simulink library "Simscape_Bit_Multiplexers_Lib"  (R2023a)
settings: Solver=ode45  StartTime=0.0  StopTime=10.0  RelTol=1e-3  EnableMultiTasking=on
libraries: Simscape_Gates_Lib x11
settings Model: Creator=uzivatel  LastModifiedBy=Jozko Mrkvicka
settings SolverCC: AlgebraicLoopSolver=TrustRegion
settings DataIOCC: LimitDataPoints=on  SaveFormat=Array  ReturnWorkspaceOutputs=off
settings OptimizationCC: LifeSpan=inf
settings DebuggingCC: UnderspecifiedInitializationDetection=Classic  MergeDetectMultiDrivingBlocksExec=none  SolverPrmCheckMsg=warning  UnconnectedInputMsg=warning  UnconnectedOutputMsg=warning  UnconnectedLineMsg=warning  StateNameClashWarn=warning  SFUnexpectedBacktrackingDiag=warning  SFNoUnconditionalDefaultTransitionDiag=warning  ArithmeticOperatorsInVariantConditions=warning
settings HardwareCC: ProdBitPerPointer=32  ProdBitPerSizeT=32  ProdBitPerPtrDiffT=32  ProdLargestAtomicFloat=None  ProdIntDivRoundTo=Undefined  ProdEndianess=Unspecified  ProdWordSize=32  ProdHWDeviceType=32-bit Generic
settings ModelReferenceCC: EnableRefExpFcnMdlSchedulingChecks=on  PropagateSignalLabelsOutOfModel=off
settings SFSimCC: SimUseLocalCustomCode=off  CustomCodeUndefinedFunction=UseInterfaceOnly
settings RTWCC: RTWUseLocalCustomCode=off
settings CodeAppCC: StateflowObjectComments=on
settings GRTTargetCC: TargetLangStandard=C89/C90 (ANSI)
settings ConfigComp: CovMetricSettings=dw  CovSaveCumulativeToWorkspaceVar=on  CovSaveSingleToWorkspaceVar=on  CovExternalEMLEnable=off

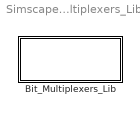
== system Simscape_Bit_Multiplexers_Lib ==
  Bit_Multiplexers_Lib : Subsystem

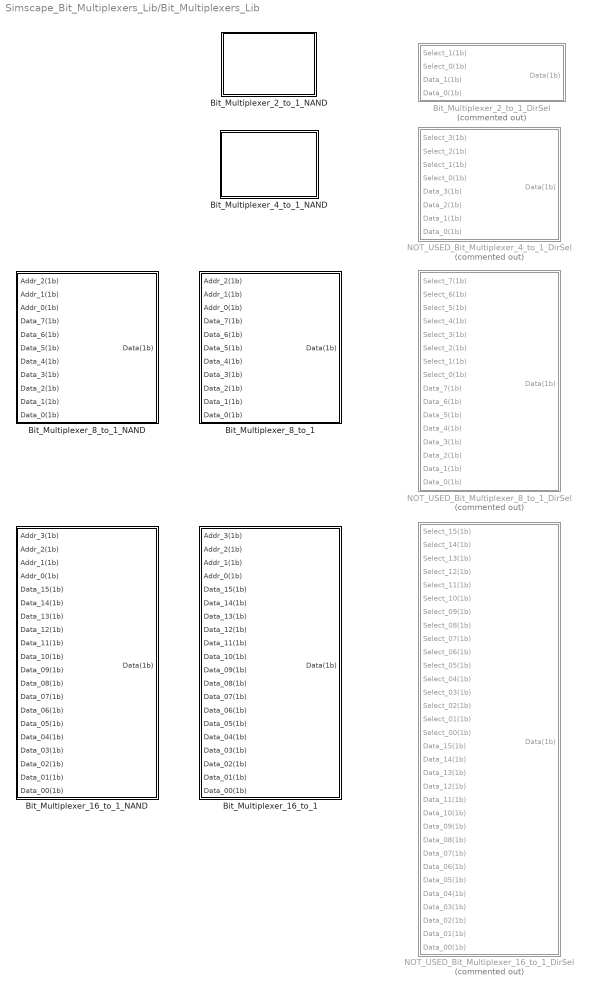
== system Simscape_Bit_Multiplexers_Lib/Bit_Multiplexers_Lib ==
  Bit_Multiplexer_16_to_1 : Subsystem
  Bit_Multiplexer_16_to_1_NAND : Subsystem
  Bit_Multiplexer_2_to_1_DirSel : Subsystem  Commented=on
  Bit_Multiplexer_2_to_1_NAND : Subsystem
      settings: PortSchema="{\"entries\":[{\"content\":{\"sides\":[{\"content\":{\"connectorIds\":[\"LConn1\",\"LConn2\",\"LConn3\"]},\"type\":\"ConnectorPlacement.EquallySpacedRectSide\",\"uuid\":\"05aa9ed7-c40b-4846-b9c5-a59fe7474fe7\"},{\"content\":{\"connectorIds\":[\"RConn1\"],\"side\":\"RIGHT\"},\"type\":\"ConnectorPlacement.EquallySpacedRectSide\",\"uuid\":\"f4c26865-c23f-4e2d-9b22-f32510006689\"},{\"content\":{\"connectorIds\":[\"LConn4\"],\"side\":\"TOP\"},\"type\":\"ConnectorPlacement.EquallySpacedRectSide\",\"uuid\":\"5ca9bb1e-e0f6-480e-8c02-f26cf148a313\"},{\"content\":{\"connectorIds\":[\"RConn2\"],\"side\":\"BOTTOM\"},\"type\":\"ConnectorPlacement.EquallySpacedRectSide\",\"uuid\":\"bd4becbe-1bbd-422f-b22f-c30d52f9b7b5\"}]},\"type\":\"ConnectorPlacement.EquallySpacedConnector\",\"uuid\":\"13373c58-d26b-438c-b680-b1e730634329\"}],\"packageUris\":[\"http://schema.mathworks.com/mf0/Connector/R2020b\"],\"version\":\"1.0\"}"
  Bit_Multiplexer_4_to_1_NAND : Subsystem
      settings: PortSchema="{\"entries\":[{\"content\":{\"sides\":[{\"content\":{\"connectorIds\":[\"LConn1\",\"LConn2\",\"LConn3\",\"LConn4\",\"LConn5\",\"LConn6\"]},\"type\":\"ConnectorPlacement.EquallySpacedRectSide\",\"uuid\":\"05aa9ed7-c40b-4846-b9c5-a59fe7474fe7\"},{\"content\":{\"connectorIds\":[\"RConn1\"],\"side\":\"RIGHT\"},\"type\":\"ConnectorPlacement.EquallySpacedRectSide\",\"uuid\":\"f4c26865-c23f-4e2d-9b22-f32510006689\"},{\"content\":{\"connectorIds\":[\"LConn7\"],\"side\":\"TOP\"},\"type\":\"ConnectorPlacement.EquallySpacedRectSide\",\"uuid\":\"5ca9bb1e-e0f6-480e-8c02-f26cf148a313\"},{\"content\":{\"connectorIds\":[\"RConn2\"],\"side\":\"BOTTOM\"},\"type\":\"ConnectorPlacement.EquallySpacedRectSide\",\"uuid\":\"bd4becbe-1bbd-422f-b22f-c30d52f9b7b5\"}]},\"type\":\"ConnectorPlacement.EquallySpacedConnector\",\"uuid\":\"13373c58-d26b-438c-b680-b1e730634329\"}],\"packageUris\":[\"http://schema.mathworks.com/mf0/Connector/R2020b\"],\"version\":\"1.0\"}"
  Bit_Multiplexer_8_to_1 : Subsystem
  Bit_Multiplexer_8_to_1_NAND : Subsystem
  NOT_USED_Bit_Multiplexer_16_to_1_DirSel : Subsystem  Commented=on
  NOT_USED_Bit_Multiplexer_4_to_1_DirSel : Subsystem  Commented=on
  NOT_USED_Bit_Multiplexer_8_to_1_DirSel : Subsystem  Commented=on

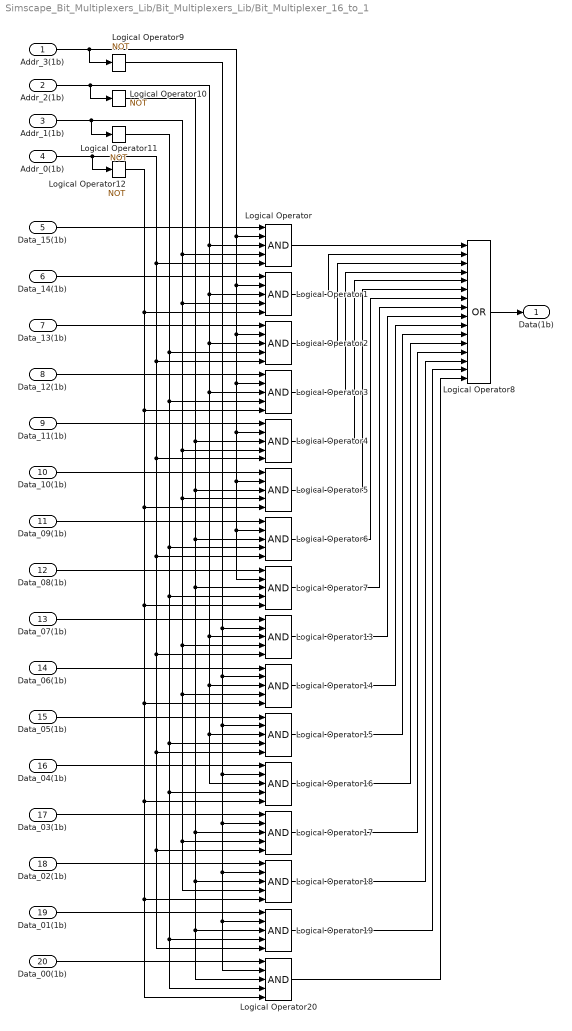
== system Simscape_Bit_Multiplexers_Lib/Bit_Multiplexers_Lib/Bit_Multiplexer_16_to_1 ==
  Addr_3(1b) : Inport
  Addr_2(1b) : Inport  Port=2
  Addr_1(1b) : Inport  Port=3
  Addr_0(1b) : Inport  Port=4
  Data_15(1b) : Inport  Port=5
  Data_14(1b) : Inport  Port=6
  Data_13(1b) : Inport  Port=7
  Data_12(1b) : Inport  Port=8
  Data_11(1b) : Inport  Port=9
  Data_10(1b) : Inport  Port=10
  Data_09(1b) : Inport  Port=11
  Data_08(1b) : Inport  Port=12
  Data_07(1b) : Inport  Port=13
  Data_06(1b) : Inport  Port=14
  Data_05(1b) : Inport  Port=15
  Data_04(1b) : Inport  Port=16
  Data_03(1b) : Inport  Port=17
  Data_02(1b) : Inport  Port=18
  Data_01(1b) : Inport  Port=19
  Data_00(1b) : Inport  Port=20
  Logical Operator{,1..7,13..20} (16 alike) : Logic  Inputs=5  IconShape=distinctive  AllPortsSameDT=off  OutDataTypeStr=boolean
  Logical Operator{9..12} (4 alike) : Logic  Operator=NOT  Inputs=4  IconShape=distinctive  AllPortsSameDT=off  OutDataTypeStr=boolean
  Logical Operator8 : Logic  Operator=OR  Inputs=16  IconShape=distinctive  OutDataTypeStr=boolean
  Data(1b) : Outport
  wires:
  Logical Operator12/1 -> Logical Operator20/5, Logical Operator18/5, Logical Operator16/5, Logical Operator14/5, Logical Operator7/5, Logical Operator5/5, Logical Operator3/5, Logical Operator1/5
  Addr_0(1b)/1 -> Logical Operator15/5, Logical Operator17/5, Logical Operator19/5, Logical Operator13/5, Logical Operator6/5, Logical Operator4/5, Logical Operator2/5, Logical Operator/5, Logical Operator12/1
  Logical Operator11/1 -> Logical Operator20/4, Logical Operator19/4, Logical Operator16/4, Logical Operator15/4, Logical Operator7/4, Logical Operator6/4, Logical Operator3/4, Logical Operator2/4
  Addr_1(1b)/1 -> Logical Operator18/4, Logical Operator17/4, Logical Operator14/4, Logical Operator13/4, Logical Operator5/4, Logical Operator4/4, Logical Operator1/4, Logical Operator/4, Logical Operator11/1
  Logical Operator10/1 -> Logical Operator20/3, Logical Operator19/3, Logical Operator18/3, Logical Operator17/3, Logical Operator7/3, Logical Operator6/3, Logical Operator5/3, Logical Operator4/3
  Addr_2(1b)/1 -> Logical Operator16/3, Logical Operator15/3, Logical Operator14/3, Logical Operator13/3, Logical Operator3/3, Logical Operator2/3, Logical Operator1/3, Logical Operator/3, Logical Operator10/1
  Logical Operator9/1 -> Logical Operator20/2, Logical Operator19/2, Logical Operator18/2, Logical Operator17/2, Logical Operator16/2, Logical Operator15/2, Logical Operator14/2, Logical Operator13/2
  Addr_3(1b)/1 -> Logical Operator3/2, Logical Operator4/2, Logical Operator7/2, Logical Operator6/2, Logical Operator5/2, Logical Operator2/2, Logical Operator1/2, Logical Operator/2, Logical Operator9/1
  Data_00(1b)/1 -> Logical Operator20/1
  Data_01(1b)/1 -> Logical Operator19/1
  Data_02(1b)/1 -> Logical Operator18/1
  Data_03(1b)/1 -> Logical Operator17/1
  Data_04(1b)/1 -> Logical Operator16/1
  Data_05(1b)/1 -> Logical Operator15/1
  Data_06(1b)/1 -> Logical Operator14/1
  Data_07(1b)/1 -> Logical Operator13/1
  Logical Operator20/1 -> Logical Operator8/16
  Logical Operator19/1 -> Logical Operator8/15
  Logical Operator18/1 -> Logical Operator8/14
  Logical Operator17/1 -> Logical Operator8/13
  Logical Operator16/1 -> Logical Operator8/12
  Logical Operator15/1 -> Logical Operator8/11
  Logical Operator14/1 -> Logical Operator8/10
  Logical Operator13/1 -> Logical Operator8/9
  Logical Operator8/1 -> Data(1b)/1
  Data_15(1b)/1 -> Logical Operator/1
  Data_14(1b)/1 -> Logical Operator1/1
  Data_13(1b)/1 -> Logical Operator2/1
  Data_12(1b)/1 -> Logical Operator3/1
  Data_11(1b)/1 -> Logical Operator4/1
  Data_10(1b)/1 -> Logical Operator5/1
  Data_09(1b)/1 -> Logical Operator6/1
  Data_08(1b)/1 -> Logical Operator7/1
  Logical Operator7/1 -> Logical Operator8/8
  Logical Operator6/1 -> Logical Operator8/7
  Logical Operator5/1 -> Logical Operator8/6
  Logical Operator4/1 -> Logical Operator8/5
  Logical Operator3/1 -> Logical Operator8/4
  Logical Operator2/1 -> Logical Operator8/3
  Logical Operator1/1 -> Logical Operator8/2
  Logical Operator/1 -> Logical Operator8/1

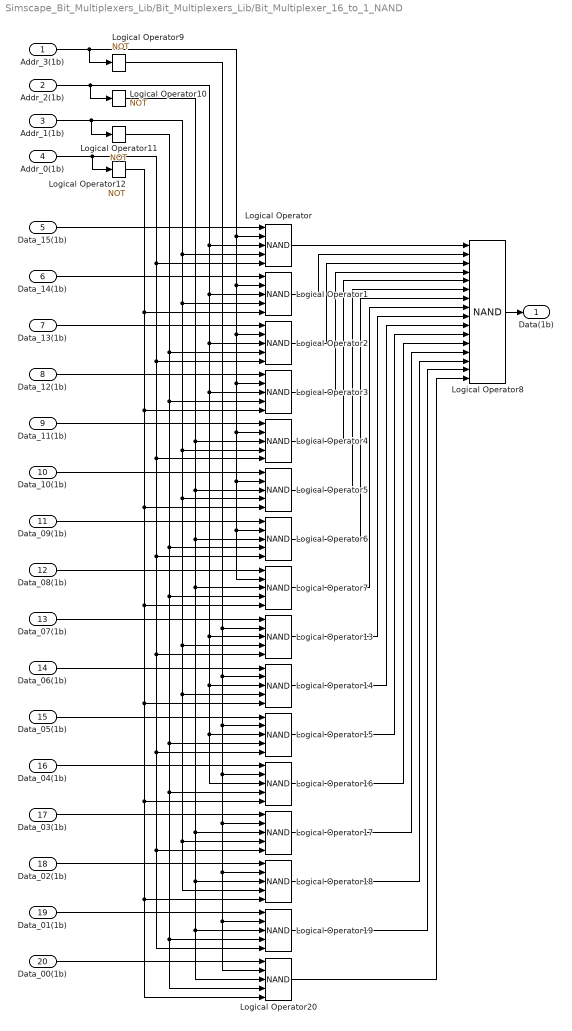
== system Simscape_Bit_Multiplexers_Lib/Bit_Multiplexers_Lib/Bit_Multiplexer_16_to_1_NAND ==
  Addr_3(1b) : Inport
  Addr_2(1b) : Inport  Port=2
  Addr_1(1b) : Inport  Port=3
  Addr_0(1b) : Inport  Port=4
  Data_15(1b) : Inport  Port=5
  Data_14(1b) : Inport  Port=6
  Data_13(1b) : Inport  Port=7
  Data_12(1b) : Inport  Port=8
  Data_11(1b) : Inport  Port=9
  Data_10(1b) : Inport  Port=10
  Data_09(1b) : Inport  Port=11
  Data_08(1b) : Inport  Port=12
  Data_07(1b) : Inport  Port=13
  Data_06(1b) : Inport  Port=14
  Data_05(1b) : Inport  Port=15
  Data_04(1b) : Inport  Port=16
  Data_03(1b) : Inport  Port=17
  Data_02(1b) : Inport  Port=18
  Data_01(1b) : Inport  Port=19
  Data_00(1b) : Inport  Port=20
  Logical Operator{,1..7,13..20} (16 alike) : Logic  Operator=NAND  Inputs=5  IconShape=distinctive  AllPortsSameDT=off  OutDataTypeStr=boolean
  Logical Operator{9..12} (4 alike) : Logic  Operator=NOT  Inputs=4  IconShape=distinctive  AllPortsSameDT=off  OutDataTypeStr=boolean
  Logical Operator8 : Logic  Operator=NAND  Inputs=16  IconShape=distinctive  OutDataTypeStr=boolean
  Data(1b) : Outport
  wires:
  Logical Operator12/1 -> Logical Operator20/5, Logical Operator18/5, Logical Operator16/5, Logical Operator14/5, Logical Operator7/5, Logical Operator5/5, Logical Operator3/5, Logical Operator1/5
  Addr_0(1b)/1 -> Logical Operator15/5, Logical Operator17/5, Logical Operator19/5, Logical Operator13/5, Logical Operator6/5, Logical Operator4/5, Logical Operator2/5, Logical Operator/5, Logical Operator12/1
  Logical Operator11/1 -> Logical Operator20/4, Logical Operator19/4, Logical Operator16/4, Logical Operator15/4, Logical Operator7/4, Logical Operator6/4, Logical Operator3/4, Logical Operator2/4
  Addr_1(1b)/1 -> Logical Operator18/4, Logical Operator17/4, Logical Operator14/4, Logical Operator13/4, Logical Operator5/4, Logical Operator4/4, Logical Operator1/4, Logical Operator/4, Logical Operator11/1
  Logical Operator10/1 -> Logical Operator20/3, Logical Operator19/3, Logical Operator18/3, Logical Operator17/3, Logical Operator7/3, Logical Operator6/3, Logical Operator5/3, Logical Operator4/3
  Addr_2(1b)/1 -> Logical Operator16/3, Logical Operator15/3, Logical Operator14/3, Logical Operator13/3, Logical Operator3/3, Logical Operator2/3, Logical Operator1/3, Logical Operator/3, Logical Operator10/1
  Logical Operator9/1 -> Logical Operator20/2, Logical Operator19/2, Logical Operator18/2, Logical Operator17/2, Logical Operator16/2, Logical Operator15/2, Logical Operator14/2, Logical Operator13/2
  Addr_3(1b)/1 -> Logical Operator3/2, Logical Operator4/2, Logical Operator7/2, Logical Operator6/2, Logical Operator5/2, Logical Operator2/2, Logical Operator1/2, Logical Operator/2, Logical Operator9/1
  Data_00(1b)/1 -> Logical Operator20/1
  Data_01(1b)/1 -> Logical Operator19/1
  Data_02(1b)/1 -> Logical Operator18/1
  Data_03(1b)/1 -> Logical Operator17/1
  Data_04(1b)/1 -> Logical Operator16/1
  Data_05(1b)/1 -> Logical Operator15/1
  Data_06(1b)/1 -> Logical Operator14/1
  Data_07(1b)/1 -> Logical Operator13/1
  Logical Operator20/1 -> Logical Operator8/16
  Logical Operator19/1 -> Logical Operator8/15
  Logical Operator18/1 -> Logical Operator8/14
  Logical Operator17/1 -> Logical Operator8/13
  Logical Operator16/1 -> Logical Operator8/12
  Logical Operator15/1 -> Logical Operator8/11
  Logical Operator14/1 -> Logical Operator8/10
  Logical Operator13/1 -> Logical Operator8/9
  Logical Operator8/1 -> Data(1b)/1
  Data_15(1b)/1 -> Logical Operator/1
  Data_14(1b)/1 -> Logical Operator1/1
  Data_13(1b)/1 -> Logical Operator2/1
  Data_12(1b)/1 -> Logical Operator3/1
  Data_11(1b)/1 -> Logical Operator4/1
  Data_10(1b)/1 -> Logical Operator5/1
  Data_09(1b)/1 -> Logical Operator6/1
  Data_08(1b)/1 -> Logical Operator7/1
  Logical Operator7/1 -> Logical Operator8/8
  Logical Operator6/1 -> Logical Operator8/7
  Logical Operator5/1 -> Logical Operator8/6
  Logical Operator4/1 -> Logical Operator8/5
  Logical Operator3/1 -> Logical Operator8/4
  Logical Operator2/1 -> Logical Operator8/3
  Logical Operator1/1 -> Logical Operator8/2
  Logical Operator/1 -> Logical Operator8/1

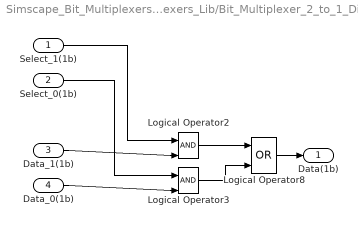
== system Simscape_Bit_Multiplexers_Lib/Bit_Multiplexers_Lib/Bit_Multiplexer_2_to_1_DirSel ==
  Select_1(1b) : Inport
  Select_0(1b) : Inport  Port=2
  Data_1(1b) : Inport  Port=3
  Data_0(1b) : Inport  Port=4
  Logical Operator2 : Logic  IconShape=distinctive  AllPortsSameDT=off  OutDataTypeStr=boolean
  Logical Operator3 : Logic  IconShape=distinctive  AllPortsSameDT=off  OutDataTypeStr=boolean
  Logical Operator8 : Logic  Operator=OR  IconShape=distinctive  OutDataTypeStr=boolean
  Data(1b) : Outport
  wires:
  Logical Operator8/1 -> Data(1b)/1
  Logical Operator3/1 -> Logical Operator8/2
  Logical Operator2/1 -> Logical Operator8/1
  Data_1(1b)/1 -> Logical Operator2/2
  Data_0(1b)/1 -> Logical Operator3/2
  Select_1(1b)/1 -> Logical Operator2/1
  Select_0(1b)/1 -> Logical Operator3/1

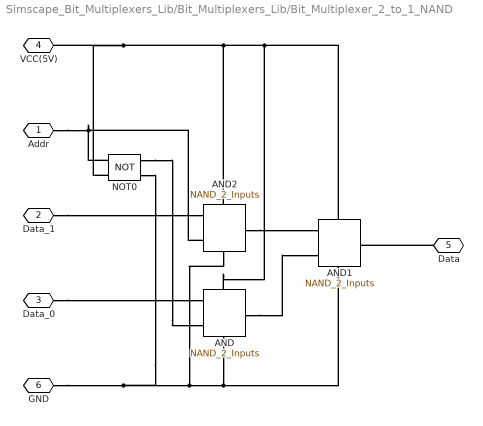
== system Simscape_Bit_Multiplexers_Lib/Bit_Multiplexers_Lib/Bit_Multiplexer_2_to_1_NAND ==
  AND : Simscape_Gates_Lib/NAND_2_Inputs  SystemSampleTime=-1  VariantActivationTime=update diagram  Latency=0  AutoFrameSizeCalculation=off
      settings: LibrarySourceBlock=pokus_lib/AND  PortSchema="{\"entries\":[{\"content\":{\"sides\":[{\"content\":{\"connectorIds\":[\"LConn1\",\"LConn2\"]},\"type\":\"ConnectorPlacement.EquallySpacedRectSide\",\"uuid\":\"1f677ca5-ee16-40a0-87d2-2e95da8c7721\"},{\"content\":{\"connectorIds\":[\"RConn1\"],\"side\":\"RIGHT\"},\"type\":\"ConnectorPlacement.EquallySpacedRectSide\",\"uuid\":\"f9e7d437-b89a-4416-b804-8f11fd927687\"},{\"content\":{\"connectorIds\":[\"LConn3\"],\"side\":\"TOP\"},\"type\":\"ConnectorPlacement.EquallySpacedRectSide\",\"uuid\":\"bd4824ff-3399-4fe5-aaaa-59980d9198b6\"},{\"content\":{\"connectorIds\":[\"RConn2\"],\"side\":\"BOTTOM\"},\"type\":\"ConnectorPlacement.EquallySpacedRectSide\",\"uuid\":\"eafb0998-9a7e-4634-b7fa-91494491415c\"}]},\"type\":\"ConnectorPlacement.EquallySpacedConnector\",\"uuid\":\"9f76a3c8-f141-459c-8f30-1ffa838c3ea4\"}],\"packageUris\":[\"http://schema.mathworks.com/mf0/Connector/R2020b\"],\"version\":\"1.0\"}"
  AND1 : Simscape_Gates_Lib/NAND_2_Inputs  SystemSampleTime=-1  VariantActivationTime=update diagram  Latency=0  AutoFrameSizeCalculation=off
      settings: LibrarySourceBlock=pokus_lib/AND  PortSchema="{\"entries\":[{\"content\":{\"sides\":[{\"content\":{\"connectorIds\":[\"LConn1\",\"LConn2\"]},\"type\":\"ConnectorPlacement.EquallySpacedRectSide\",\"uuid\":\"1f677ca5-ee16-40a0-87d2-2e95da8c7721\"},{\"content\":{\"connectorIds\":[\"RConn1\"],\"side\":\"RIGHT\"},\"type\":\"ConnectorPlacement.EquallySpacedRectSide\",\"uuid\":\"f9e7d437-b89a-4416-b804-8f11fd927687\"},{\"content\":{\"connectorIds\":[\"LConn3\"],\"side\":\"TOP\"},\"type\":\"ConnectorPlacement.EquallySpacedRectSide\",\"uuid\":\"bd4824ff-3399-4fe5-aaaa-59980d9198b6\"},{\"content\":{\"connectorIds\":[\"RConn2\"],\"side\":\"BOTTOM\"},\"type\":\"ConnectorPlacement.EquallySpacedRectSide\",\"uuid\":\"eafb0998-9a7e-4634-b7fa-91494491415c\"}]},\"type\":\"ConnectorPlacement.EquallySpacedConnector\",\"uuid\":\"9f76a3c8-f141-459c-8f30-1ffa838c3ea4\"}],\"packageUris\":[\"http://schema.mathworks.com/mf0/Connector/R2020b\"],\"version\":\"1.0\"}"
  AND2 : Simscape_Gates_Lib/NAND_2_Inputs  SystemSampleTime=-1  VariantActivationTime=update diagram  Latency=0  AutoFrameSizeCalculation=off
      settings: LibrarySourceBlock=pokus_lib/AND  PortSchema="{\"entries\":[{\"content\":{\"sides\":[{\"content\":{\"connectorIds\":[\"LConn1\",\"LConn2\"]},\"type\":\"ConnectorPlacement.EquallySpacedRectSide\",\"uuid\":\"1f677ca5-ee16-40a0-87d2-2e95da8c7721\"},{\"content\":{\"connectorIds\":[\"RConn1\"],\"side\":\"RIGHT\"},\"type\":\"ConnectorPlacement.EquallySpacedRectSide\",\"uuid\":\"f9e7d437-b89a-4416-b804-8f11fd927687\"},{\"content\":{\"connectorIds\":[\"LConn3\"],\"side\":\"TOP\"},\"type\":\"ConnectorPlacement.EquallySpacedRectSide\",\"uuid\":\"bd4824ff-3399-4fe5-aaaa-59980d9198b6\"},{\"content\":{\"connectorIds\":[\"RConn2\"],\"side\":\"BOTTOM\"},\"type\":\"ConnectorPlacement.EquallySpacedRectSide\",\"uuid\":\"eafb0998-9a7e-4634-b7fa-91494491415c\"}]},\"type\":\"ConnectorPlacement.EquallySpacedConnector\",\"uuid\":\"9f76a3c8-f141-459c-8f30-1ffa838c3ea4\"}],\"packageUris\":[\"http://schema.mathworks.com/mf0/Connector/R2020b\"],\"version\":\"1.0\"}"
  NOT0 : Simscape_Gates_Lib/NOT
  Addr : PMIOPort  Side=Left
  Data_1 : PMIOPort  Port=2  Side=Left
  Data_0 : PMIOPort  Port=3  Side=Left
  VCC(5V) : PMIOPort  Port=4  Side=Left
  Data : PMIOPort  Port=5  Side=Right
  GND : PMIOPort  Port=6  Side=Right
  connections:
  VCC(5V)/RConn1 -- AND2/LConn3 -- AND1/LConn3 -- AND/LConn3 -- NOT0/LConn2
  Data_0/RConn1 -- AND/LConn1
  Data_1/RConn1 -- AND2/LConn1
  NOT0/RConn1 -- AND/LConn2
  AND2/RConn1 -- AND1/LConn1
  AND/RConn1 -- AND1/LConn2
  Data/RConn1 -- AND1/RConn1
  AND2/LConn2 -- Addr/RConn1 -- NOT0/LConn1
  AND/RConn2 -- AND1/RConn2 -- AND2/RConn2 -- GND/RConn1 -- NOT0/RConn2

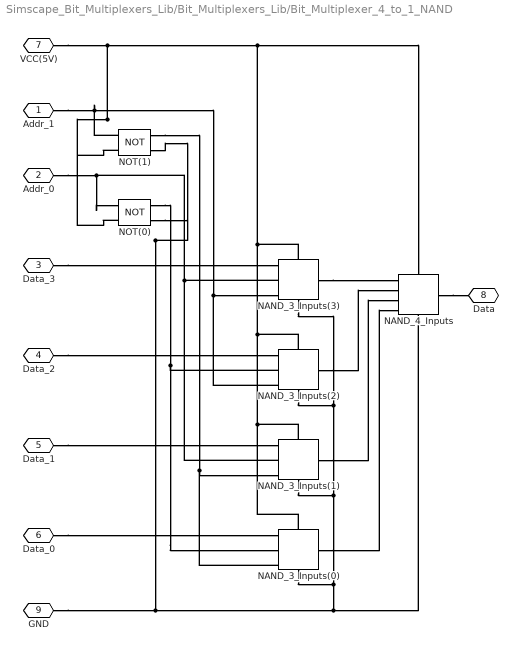
== system Simscape_Bit_Multiplexers_Lib/Bit_Multiplexers_Lib/Bit_Multiplexer_4_to_1_NAND ==
  NAND_3_Inputs(0) : Simscape_Gates_Lib/NAND_3_Inputs  SystemSampleTime=-1  VariantActivationTime=update diagram  Latency=0  AutoFrameSizeCalculation=off
      settings: PortSchema="{\"entries\":[{\"content\":{\"sides\":[{\"content\":{\"connectorIds\":[\"LConn1\",\"LConn2\",\"LConn3\"]},\"type\":\"ConnectorPlacement.EquallySpacedRectSide\",\"uuid\":\"3ad033e8-f540-4908-b767-0851e4a6512c\"},{\"content\":{\"connectorIds\":[\"RConn1\"],\"side\":\"RIGHT\"},\"type\":\"ConnectorPlacement.EquallySpacedRectSide\",\"uuid\":\"66ead7bd-a472-46db-941e-d4ec7399d328\"},{\"content\":{\"connectorIds\":[\"LConn4\"],\"side\":\"TOP\"},\"type\":\"ConnectorPlacement.EquallySpacedRectSide\",\"uuid\":\"cb3c8fc5-feff-4b6f-b91b-692680a0eeb1\"},{\"content\":{\"connectorIds\":[\"RConn2\"],\"side\":\"BOTTOM\"},\"type\":\"ConnectorPlacement.EquallySpacedRectSide\",\"uuid\":\"f8b8aaf7-b6fc-45dd-a5cf-24360dfeaf9c\"}]},\"type\":\"ConnectorPlacement.EquallySpacedConnector\",\"uuid\":\"2d561a3f-f784-4d92-a395-6823d790bdb8\"}],\"packageUris\":[\"http://schema.mathworks.com/mf0/Connector/R2020b\"],\"version\":\"1.0\"}"
  NAND_3_Inputs(1) : Simscape_Gates_Lib/NAND_3_Inputs  SystemSampleTime=-1  VariantActivationTime=update diagram  Latency=0  AutoFrameSizeCalculation=off
      settings: PortSchema="{\"entries\":[{\"content\":{\"sides\":[{\"content\":{\"connectorIds\":[\"LConn1\",\"LConn2\",\"LConn3\"]},\"type\":\"ConnectorPlacement.EquallySpacedRectSide\",\"uuid\":\"3ad033e8-f540-4908-b767-0851e4a6512c\"},{\"content\":{\"connectorIds\":[\"RConn1\"],\"side\":\"RIGHT\"},\"type\":\"ConnectorPlacement.EquallySpacedRectSide\",\"uuid\":\"66ead7bd-a472-46db-941e-d4ec7399d328\"},{\"content\":{\"connectorIds\":[\"LConn4\"],\"side\":\"TOP\"},\"type\":\"ConnectorPlacement.EquallySpacedRectSide\",\"uuid\":\"cb3c8fc5-feff-4b6f-b91b-692680a0eeb1\"},{\"content\":{\"connectorIds\":[\"RConn2\"],\"side\":\"BOTTOM\"},\"type\":\"ConnectorPlacement.EquallySpacedRectSide\",\"uuid\":\"f8b8aaf7-b6fc-45dd-a5cf-24360dfeaf9c\"}]},\"type\":\"ConnectorPlacement.EquallySpacedConnector\",\"uuid\":\"2d561a3f-f784-4d92-a395-6823d790bdb8\"}],\"packageUris\":[\"http://schema.mathworks.com/mf0/Connector/R2020b\"],\"version\":\"1.0\"}"
  NAND_3_Inputs(2) : Simscape_Gates_Lib/NAND_3_Inputs  SystemSampleTime=-1  VariantActivationTime=update diagram  Latency=0  AutoFrameSizeCalculation=off
      settings: PortSchema="{\"entries\":[{\"content\":{\"sides\":[{\"content\":{\"connectorIds\":[\"LConn1\",\"LConn2\",\"LConn3\"]},\"type\":\"ConnectorPlacement.EquallySpacedRectSide\",\"uuid\":\"3ad033e8-f540-4908-b767-0851e4a6512c\"},{\"content\":{\"connectorIds\":[\"RConn1\"],\"side\":\"RIGHT\"},\"type\":\"ConnectorPlacement.EquallySpacedRectSide\",\"uuid\":\"66ead7bd-a472-46db-941e-d4ec7399d328\"},{\"content\":{\"connectorIds\":[\"LConn4\"],\"side\":\"TOP\"},\"type\":\"ConnectorPlacement.EquallySpacedRectSide\",\"uuid\":\"cb3c8fc5-feff-4b6f-b91b-692680a0eeb1\"},{\"content\":{\"connectorIds\":[\"RConn2\"],\"side\":\"BOTTOM\"},\"type\":\"ConnectorPlacement.EquallySpacedRectSide\",\"uuid\":\"f8b8aaf7-b6fc-45dd-a5cf-24360dfeaf9c\"}]},\"type\":\"ConnectorPlacement.EquallySpacedConnector\",\"uuid\":\"2d561a3f-f784-4d92-a395-6823d790bdb8\"}],\"packageUris\":[\"http://schema.mathworks.com/mf0/Connector/R2020b\"],\"version\":\"1.0\"}"
  NAND_3_Inputs(3) : Simscape_Gates_Lib/NAND_3_Inputs  SystemSampleTime=-1  VariantActivationTime=update diagram  Latency=0  AutoFrameSizeCalculation=off
      settings: PortSchema="{\"entries\":[{\"content\":{\"sides\":[{\"content\":{\"connectorIds\":[\"LConn1\",\"LConn2\",\"LConn3\"]},\"type\":\"ConnectorPlacement.EquallySpacedRectSide\",\"uuid\":\"3ad033e8-f540-4908-b767-0851e4a6512c\"},{\"content\":{\"connectorIds\":[\"RConn1\"],\"side\":\"RIGHT\"},\"type\":\"ConnectorPlacement.EquallySpacedRectSide\",\"uuid\":\"66ead7bd-a472-46db-941e-d4ec7399d328\"},{\"content\":{\"connectorIds\":[\"LConn4\"],\"side\":\"TOP\"},\"type\":\"ConnectorPlacement.EquallySpacedRectSide\",\"uuid\":\"cb3c8fc5-feff-4b6f-b91b-692680a0eeb1\"},{\"content\":{\"connectorIds\":[\"RConn2\"],\"side\":\"BOTTOM\"},\"type\":\"ConnectorPlacement.EquallySpacedRectSide\",\"uuid\":\"f8b8aaf7-b6fc-45dd-a5cf-24360dfeaf9c\"}]},\"type\":\"ConnectorPlacement.EquallySpacedConnector\",\"uuid\":\"2d561a3f-f784-4d92-a395-6823d790bdb8\"}],\"packageUris\":[\"http://schema.mathworks.com/mf0/Connector/R2020b\"],\"version\":\"1.0\"}"
  NAND_4_Inputs : Simscape_Gates_Lib/NAND_4_Inputs  SystemSampleTime=-1  VariantActivationTime=update diagram  Latency=0  AutoFrameSizeCalculation=off
      settings: PortSchema="{\"entries\":[{\"content\":{\"sides\":[{\"content\":{\"connectorIds\":[\"LConn1\",\"LConn2\",\"LConn3\",\"LConn4\"]},\"type\":\"ConnectorPlacement.EquallySpacedRectSide\",\"uuid\":\"4919ea86-d7f6-40d9-8c6d-90ddc4d67a92\"},{\"content\":{\"connectorIds\":[\"RConn1\"],\"side\":\"RIGHT\"},\"type\":\"ConnectorPlacement.EquallySpacedRectSide\",\"uuid\":\"1df2866f-d4b5-4a77-86de-714a74631175\"},{\"content\":{\"connectorIds\":[\"LConn5\"],\"side\":\"TOP\"},\"type\":\"ConnectorPlacement.EquallySpacedRectSide\",\"uuid\":\"d2ff5589-d2f7-4904-bc04-37eddab71799\"},{\"content\":{\"connectorIds\":[\"RConn2\"],\"side\":\"BOTTOM\"},\"type\":\"ConnectorPlacement.EquallySpacedRectSide\",\"uuid\":\"d97c62b3-511d-41ae-a18a-ca90ba3cee24\"}]},\"type\":\"ConnectorPlacement.EquallySpacedConnector\",\"uuid\":\"361286e1-4e89-40b7-926b-afe9d68e3bc9\"}],\"packageUris\":[\"http://schema.mathworks.com/mf0/Connector/R2020b\"],\"version\":\"1.0\"}"
  NOT(0) : Simscape_Gates_Lib/NOT
  NOT(1) : Simscape_Gates_Lib/NOT
  Addr_1 : PMIOPort  Side=Left
  Addr_0 : PMIOPort  Port=2  Side=Left
  Data_3 : PMIOPort  Port=3  Side=Left
  Data_2 : PMIOPort  Port=4  Side=Left
  Data_1 : PMIOPort  Port=5  Side=Left
  Data_0 : PMIOPort  Port=6  Side=Left
  VCC(5V) : PMIOPort  Port=7  Side=Left
  Data : PMIOPort  Port=8  Side=Right
  GND : PMIOPort  Port=9  Side=Right
  connections:
  NAND_4_Inputs/RConn1 -- Data/RConn1
  NAND_3_Inputs(3)/RConn1 -- NAND_4_Inputs/LConn1
  NAND_3_Inputs(2)/RConn1 -- NAND_4_Inputs/LConn2
  NAND_3_Inputs(1)/RConn1 -- NAND_4_Inputs/LConn3
  NAND_3_Inputs(0)/RConn1 -- NAND_4_Inputs/LConn4
  NOT(0)/RConn1 -- NAND_3_Inputs(2)/LConn2 -- NAND_3_Inputs(0)/LConn2
  NAND_3_Inputs(3)/LConn2 -- NAND_3_Inputs(1)/LConn2 -- NOT(0)/LConn1 -- Addr_0/RConn1
  Addr_1/RConn1 -- NOT(1)/LConn1 -- NAND_3_Inputs(3)/LConn3 -- NAND_3_Inputs(2)/LConn3
  NOT(1)/RConn1 -- NAND_3_Inputs(1)/LConn3 -- NAND_3_Inputs(0)/LConn3
  Data_3/RConn1 -- NAND_3_Inputs(3)/LConn1
  Data_2/RConn1 -- NAND_3_Inputs(2)/LConn1
  Data_1/RConn1 -- NAND_3_Inputs(1)/LConn1
  Data_0/RConn1 -- NAND_3_Inputs(0)/LConn1
  VCC(5V)/RConn1 -- NOT(0)/LConn2 -- NOT(1)/LConn2 -- NAND_3_Inputs(0)/LConn4 -- NAND_3_Inputs(1)/LConn4 -- NAND_3_Inputs(2)/LConn4 -- NAND_3_Inputs(3)/LConn4 -- NAND_4_Inputs/LConn5
  GND/RConn1 -- NOT(0)/RConn2 -- NOT(1)/RConn2 -- NAND_3_Inputs(2)/RConn2 -- NAND_3_Inputs(3)/RConn2 -- NAND_3_Inputs(1)/RConn2 -- NAND_3_Inputs(0)/RConn2 -- NAND_4_Inputs/RConn2

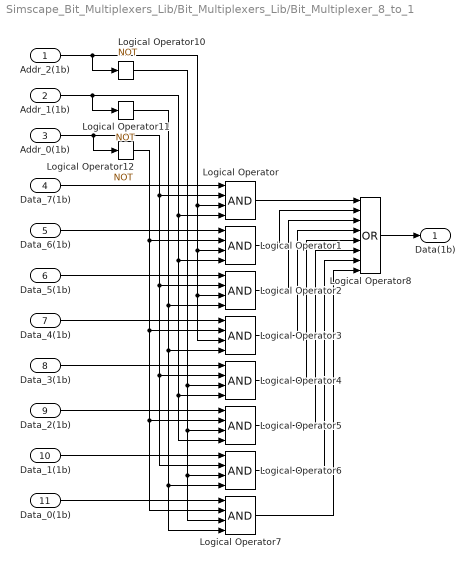
== system Simscape_Bit_Multiplexers_Lib/Bit_Multiplexers_Lib/Bit_Multiplexer_8_to_1 ==
  Addr_2(1b) : Inport
  Addr_1(1b) : Inport  Port=2
  Addr_0(1b) : Inport  Port=3
  Data_7(1b) : Inport  Port=4
  Data_6(1b) : Inport  Port=5
  Data_5(1b) : Inport  Port=6
  Data_4(1b) : Inport  Port=7
  Data_3(1b) : Inport  Port=8
  Data_2(1b) : Inport  Port=9
  Data_1(1b) : Inport  Port=10
  Data_0(1b) : Inport  Port=11
  Logical Operator{,1..7} (8 alike) : Logic  Inputs=4  IconShape=distinctive  AllPortsSameDT=off  OutDataTypeStr=boolean
  Logical Operator10 : Logic  Operator=NOT  Inputs=4  IconShape=distinctive  AllPortsSameDT=off  OutDataTypeStr=boolean
  Logical Operator11 : Logic  Operator=NOT  Inputs=4  IconShape=distinctive  AllPortsSameDT=off  OutDataTypeStr=boolean
  Logical Operator12 : Logic  Operator=NOT  Inputs=4  IconShape=distinctive  AllPortsSameDT=off  OutDataTypeStr=boolean
  Logical Operator8 : Logic  Operator=OR  Inputs=8  IconShape=distinctive  OutDataTypeStr=boolean
  Data(1b) : Outport
  wires:
  Logical Operator12/1 -> Logical Operator7/2, Logical Operator5/2, Logical Operator3/2, Logical Operator1/2
  Addr_0(1b)/1 -> Logical Operator12/1, Logical Operator6/2, Logical Operator4/2, Logical Operator2/2, Logical Operator/2
  Logical Operator11/1 -> Logical Operator7/4, Logical Operator6/4, Logical Operator3/4, Logical Operator2/4
  Addr_1(1b)/1 -> Logical Operator11/1, Logical Operator5/4, Logical Operator4/4, Logical Operator1/4, Logical Operator/4
  Logical Operator10/1 -> Logical Operator7/3, Logical Operator6/3, Logical Operator5/3, Logical Operator4/3
  Addr_2(1b)/1 -> Logical Operator3/3, Logical Operator2/3, Logical Operator1/3, Logical Operator/3, Logical Operator10/1
  Logical Operator8/1 -> Data(1b)/1
  Data_7(1b)/1 -> Logical Operator/1
  Data_6(1b)/1 -> Logical Operator1/1
  Data_5(1b)/1 -> Logical Operator2/1
  Data_4(1b)/1 -> Logical Operator3/1
  Data_3(1b)/1 -> Logical Operator4/1
  Data_2(1b)/1 -> Logical Operator5/1
  Data_1(1b)/1 -> Logical Operator6/1
  Data_0(1b)/1 -> Logical Operator7/1
  Logical Operator7/1 -> Logical Operator8/8
  Logical Operator6/1 -> Logical Operator8/7
  Logical Operator5/1 -> Logical Operator8/6
  Logical Operator4/1 -> Logical Operator8/5
  Logical Operator3/1 -> Logical Operator8/4
  Logical Operator2/1 -> Logical Operator8/3
  Logical Operator1/1 -> Logical Operator8/2
  Logical Operator/1 -> Logical Operator8/1

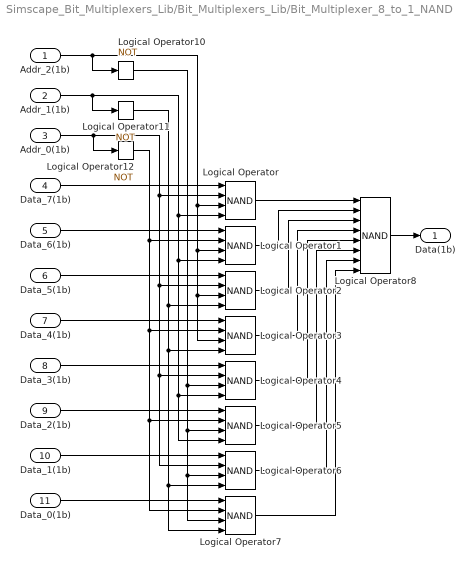
== system Simscape_Bit_Multiplexers_Lib/Bit_Multiplexers_Lib/Bit_Multiplexer_8_to_1_NAND ==
  Addr_2(1b) : Inport
  Addr_1(1b) : Inport  Port=2
  Addr_0(1b) : Inport  Port=3
  Data_7(1b) : Inport  Port=4
  Data_6(1b) : Inport  Port=5
  Data_5(1b) : Inport  Port=6
  Data_4(1b) : Inport  Port=7
  Data_3(1b) : Inport  Port=8
  Data_2(1b) : Inport  Port=9
  Data_1(1b) : Inport  Port=10
  Data_0(1b) : Inport  Port=11
  Logical Operator{,1..7} (8 alike) : Logic  Operator=NAND  Inputs=4  IconShape=distinctive  AllPortsSameDT=off  OutDataTypeStr=boolean
  Logical Operator10 : Logic  Operator=NOT  Inputs=4  IconShape=distinctive  AllPortsSameDT=off  OutDataTypeStr=boolean
  Logical Operator11 : Logic  Operator=NOT  Inputs=4  IconShape=distinctive  AllPortsSameDT=off  OutDataTypeStr=boolean
  Logical Operator12 : Logic  Operator=NOT  Inputs=4  IconShape=distinctive  AllPortsSameDT=off  OutDataTypeStr=boolean
  Logical Operator8 : Logic  Operator=NAND  Inputs=8  IconShape=distinctive  OutDataTypeStr=boolean
  Data(1b) : Outport
  wires:
  Logical Operator12/1 -> Logical Operator7/2, Logical Operator5/2, Logical Operator3/2, Logical Operator1/2
  Addr_0(1b)/1 -> Logical Operator12/1, Logical Operator6/2, Logical Operator4/2, Logical Operator2/2, Logical Operator/2
  Logical Operator11/1 -> Logical Operator7/4, Logical Operator6/4, Logical Operator3/4, Logical Operator2/4
  Addr_1(1b)/1 -> Logical Operator11/1, Logical Operator5/4, Logical Operator4/4, Logical Operator1/4, Logical Operator/4
  Logical Operator10/1 -> Logical Operator7/3, Logical Operator6/3, Logical Operator5/3, Logical Operator4/3
  Addr_2(1b)/1 -> Logical Operator3/3, Logical Operator2/3, Logical Operator1/3, Logical Operator/3, Logical Operator10/1
  Logical Operator8/1 -> Data(1b)/1
  Data_7(1b)/1 -> Logical Operator/1
  Data_6(1b)/1 -> Logical Operator1/1
  Data_5(1b)/1 -> Logical Operator2/1
  Data_4(1b)/1 -> Logical Operator3/1
  Data_3(1b)/1 -> Logical Operator4/1
  Data_2(1b)/1 -> Logical Operator5/1
  Data_1(1b)/1 -> Logical Operator6/1
  Data_0(1b)/1 -> Logical Operator7/1
  Logical Operator7/1 -> Logical Operator8/8
  Logical Operator6/1 -> Logical Operator8/7
  Logical Operator5/1 -> Logical Operator8/6
  Logical Operator4/1 -> Logical Operator8/5
  Logical Operator3/1 -> Logical Operator8/4
  Logical Operator2/1 -> Logical Operator8/3
  Logical Operator1/1 -> Logical Operator8/2
  Logical Operator/1 -> Logical Operator8/1

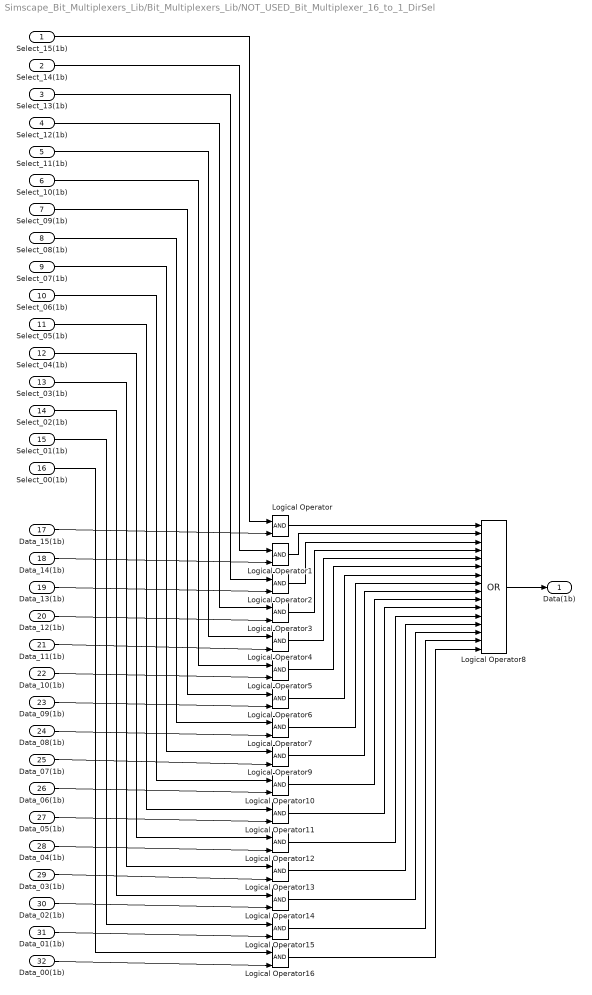
== system Simscape_Bit_Multiplexers_Lib/Bit_Multiplexers_Lib/NOT_USED_Bit_Multiplexer_16_to_1_DirSel ==
  Select_15(1b) : Inport
  Select_14(1b) : Inport  Port=2
  Select_13(1b) : Inport  Port=3
  Select_12(1b) : Inport  Port=4
  Select_11(1b) : Inport  Port=5
  Select_10(1b) : Inport  Port=6
  Select_09(1b) : Inport  Port=7
  Select_08(1b) : Inport  Port=8
  Select_07(1b) : Inport  Port=9
  Select_06(1b) : Inport  Port=10
  Select_05(1b) : Inport  Port=11
  Select_04(1b) : Inport  Port=12
  Select_03(1b) : Inport  Port=13
  Select_02(1b) : Inport  Port=14
  Select_01(1b) : Inport  Port=15
  Select_00(1b) : Inport  Port=16
  Data_15(1b) : Inport  Port=17
  Data_14(1b) : Inport  Port=18
  Data_13(1b) : Inport  Port=19
  Data_12(1b) : Inport  Port=20
  Data_11(1b) : Inport  Port=21
  Data_10(1b) : Inport  Port=22
  Data_09(1b) : Inport  Port=23
  Data_08(1b) : Inport  Port=24
  Data_07(1b) : Inport  Port=25
  Data_06(1b) : Inport  Port=26
  Data_05(1b) : Inport  Port=27
  Data_04(1b) : Inport  Port=28
  Data_03(1b) : Inport  Port=29
  Data_02(1b) : Inport  Port=30
  Data_01(1b) : Inport  Port=31
  Data_00(1b) : Inport  Port=32
  Logical Operator{,1..7,9..16} (16 alike) : Logic  IconShape=distinctive  AllPortsSameDT=off  OutDataTypeStr=boolean
  Logical Operator8 : Logic  Operator=OR  Inputs=16  IconShape=distinctive  OutDataTypeStr=boolean
  Data(1b) : Outport
  wires:
  Logical Operator8/1 -> Data(1b)/1
  Logical Operator3/1 -> Logical Operator8/4
  Logical Operator2/1 -> Logical Operator8/3
  Logical Operator1/1 -> Logical Operator8/2
  Logical Operator/1 -> Logical Operator8/1
  Data_15(1b)/1 -> Logical Operator/2
  Data_14(1b)/1 -> Logical Operator1/2
  Data_13(1b)/1 -> Logical Operator2/2
  Data_12(1b)/1 -> Logical Operator3/2
  Select_15(1b)/1 -> Logical Operator/1
  Select_14(1b)/1 -> Logical Operator1/1
  Select_13(1b)/1 -> Logical Operator2/1
  Select_12(1b)/1 -> Logical Operator3/1
  Logical Operator7/1 -> Logical Operator8/8
  Logical Operator6/1 -> Logical Operator8/7
  Logical Operator5/1 -> Logical Operator8/6
  Logical Operator4/1 -> Logical Operator8/5
  Data_11(1b)/1 -> Logical Operator4/2
  Data_10(1b)/1 -> Logical Operator5/2
  Data_09(1b)/1 -> Logical Operator6/2
  Data_08(1b)/1 -> Logical Operator7/2
  Select_11(1b)/1 -> Logical Operator4/1
  Select_10(1b)/1 -> Logical Operator5/1
  Select_09(1b)/1 -> Logical Operator6/1
  Select_08(1b)/1 -> Logical Operator7/1
  Logical Operator12/1 -> Logical Operator8/12
  Logical Operator11/1 -> Logical Operator8/11
  Logical Operator10/1 -> Logical Operator8/10
  Logical Operator9/1 -> Logical Operator8/9
  Data_07(1b)/1 -> Logical Operator9/2
  Data_06(1b)/1 -> Logical Operator10/2
  Data_05(1b)/1 -> Logical Operator11/2
  Data_04(1b)/1 -> Logical Operator12/2
  Select_07(1b)/1 -> Logical Operator9/1
  Select_06(1b)/1 -> Logical Operator10/1
  Select_05(1b)/1 -> Logical Operator11/1
  Select_04(1b)/1 -> Logical Operator12/1
  Logical Operator16/1 -> Logical Operator8/16
  Logical Operator15/1 -> Logical Operator8/15
  Logical Operator14/1 -> Logical Operator8/14
  Logical Operator13/1 -> Logical Operator8/13
  Data_03(1b)/1 -> Logical Operator13/2
  Data_02(1b)/1 -> Logical Operator14/2
  Data_01(1b)/1 -> Logical Operator15/2
  Data_00(1b)/1 -> Logical Operator16/2
  Select_03(1b)/1 -> Logical Operator13/1
  Select_02(1b)/1 -> Logical Operator14/1
  Select_01(1b)/1 -> Logical Operator15/1
  Select_00(1b)/1 -> Logical Operator16/1

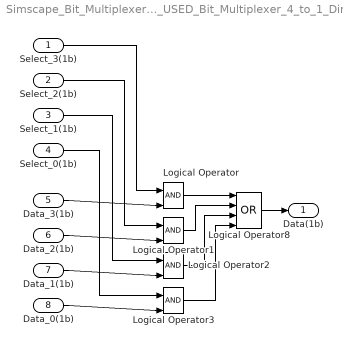
== system Simscape_Bit_Multiplexers_Lib/Bit_Multiplexers_Lib/NOT_USED_Bit_Multiplexer_4_to_1_DirSel ==
  Select_3(1b) : Inport
  Select_2(1b) : Inport  Port=2
  Select_1(1b) : Inport  Port=3
  Select_0(1b) : Inport  Port=4
  Data_3(1b) : Inport  Port=5
  Data_2(1b) : Inport  Port=6
  Data_1(1b) : Inport  Port=7
  Data_0(1b) : Inport  Port=8
  Logical Operator{,1..3} (4 alike) : Logic  IconShape=distinctive  AllPortsSameDT=off  OutDataTypeStr=boolean
  Logical Operator8 : Logic  Operator=OR  Inputs=4  IconShape=distinctive  OutDataTypeStr=boolean
  Data(1b) : Outport
  wires:
  Logical Operator8/1 -> Data(1b)/1
  Logical Operator3/1 -> Logical Operator8/4
  Logical Operator2/1 -> Logical Operator8/3
  Logical Operator1/1 -> Logical Operator8/2
  Logical Operator/1 -> Logical Operator8/1
  Data_3(1b)/1 -> Logical Operator/2
  Data_2(1b)/1 -> Logical Operator1/2
  Data_1(1b)/1 -> Logical Operator2/2
  Data_0(1b)/1 -> Logical Operator3/2
  Select_3(1b)/1 -> Logical Operator/1
  Select_2(1b)/1 -> Logical Operator1/1
  Select_1(1b)/1 -> Logical Operator2/1
  Select_0(1b)/1 -> Logical Operator3/1

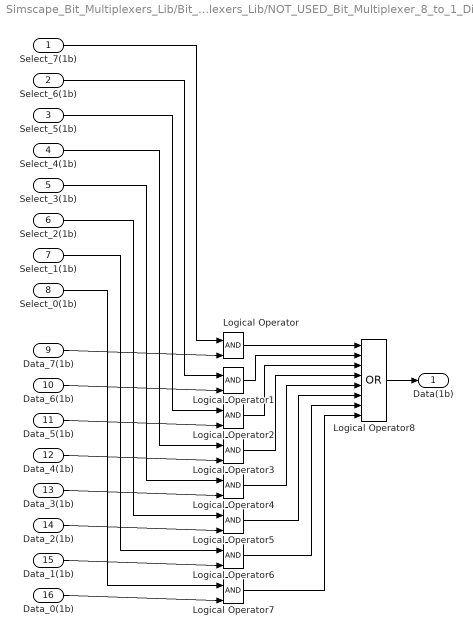
== system Simscape_Bit_Multiplexers_Lib/Bit_Multiplexers_Lib/NOT_USED_Bit_Multiplexer_8_to_1_DirSel ==
  Select_7(1b) : Inport
  Select_6(1b) : Inport  Port=2
  Select_5(1b) : Inport  Port=3
  Select_4(1b) : Inport  Port=4
  Select_3(1b) : Inport  Port=5
  Select_2(1b) : Inport  Port=6
  Select_1(1b) : Inport  Port=7
  Select_0(1b) : Inport  Port=8
  Data_7(1b) : Inport  Port=9
  Data_6(1b) : Inport  Port=10
  Data_5(1b) : Inport  Port=11
  Data_4(1b) : Inport  Port=12
  Data_3(1b) : Inport  Port=13
  Data_2(1b) : Inport  Port=14
  Data_1(1b) : Inport  Port=15
  Data_0(1b) : Inport  Port=16
  Logical Operator{,1..7} (8 alike) : Logic  IconShape=distinctive  AllPortsSameDT=off  OutDataTypeStr=boolean
  Logical Operator8 : Logic  Operator=OR  Inputs=8  IconShape=distinctive  OutDataTypeStr=boolean
  Data(1b) : Outport
  wires:
  Logical Operator8/1 -> Data(1b)/1
  Logical Operator3/1 -> Logical Operator8/4
  Logical Operator2/1 -> Logical Operator8/3
  Logical Operator1/1 -> Logical Operator8/2
  Logical Operator/1 -> Logical Operator8/1
  Data_7(1b)/1 -> Logical Operator/2
  Data_6(1b)/1 -> Logical Operator1/2
  Data_5(1b)/1 -> Logical Operator2/2
  Data_4(1b)/1 -> Logical Operator3/2
  Select_7(1b)/1 -> Logical Operator/1
  Select_6(1b)/1 -> Logical Operator1/1
  Select_5(1b)/1 -> Logical Operator2/1
  Select_4(1b)/1 -> Logical Operator3/1
  Logical Operator7/1 -> Logical Operator8/8
  Logical Operator6/1 -> Logical Operator8/7
  Logical Operator5/1 -> Logical Operator8/6
  Logical Operator4/1 -> Logical Operator8/5
  Data_3(1b)/1 -> Logical Operator4/2
  Data_2(1b)/1 -> Logical Operator5/2
  Data_1(1b)/1 -> Logical Operator6/2
  Data_0(1b)/1 -> Logical Operator7/2
  Select_3(1b)/1 -> Logical Operator4/1
  Select_2(1b)/1 -> Logical Operator5/1
  Select_1(1b)/1 -> Logical Operator6/1
  Select_0(1b)/1 -> Logical Operator7/1
